simulink model "Laptime_Simulation"  (R2020a)
settings: Solver=VariableStepAuto  StartTime=0.0  StopTime=10.0  RelTol=1e-3
model workspace (MAT data in the model file):
  A = 2
undefined symbols (not defined in the file or in its folder): m_ges
libraries: autolibshared x1
settings Model: Creator=eunde  LastModifiedBy=eunde

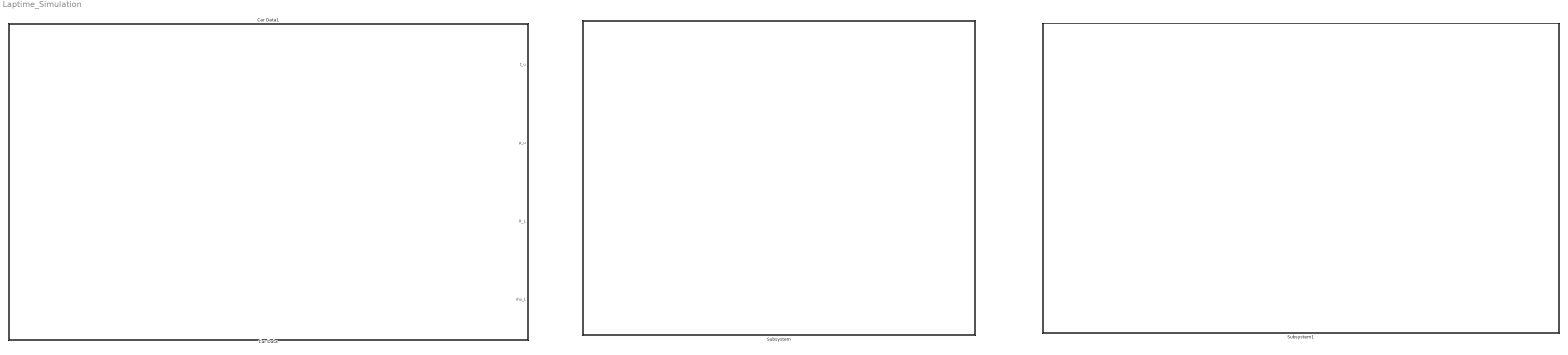
== system Laptime_Simulation ==
  Car Data : Subsystem
  Car Data1 : Subsystem
  Subsystem : Subsystem
  Subsystem1 : Subsystem

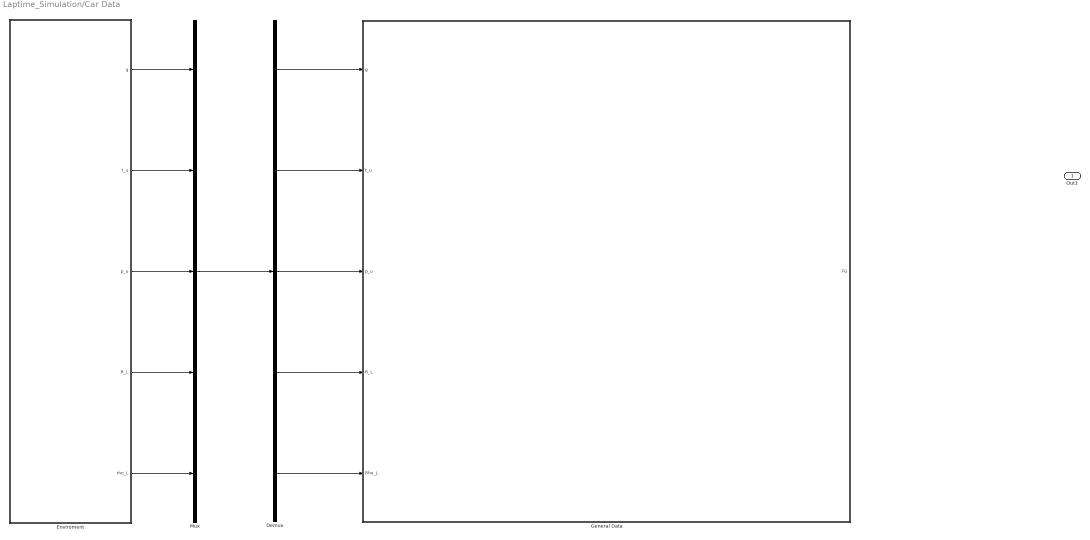
== system Laptime_Simulation/Car Data ==
  Demux : Demux  Outputs=5
  Enviroment : Subsystem
  General Data : Subsystem
  Mux : Mux  Inputs=5
  Out1 : Outport
  wires:
  Enviroment/1(g) -> Mux/1
  Enviroment/2(t_u) -> Mux/2
  Enviroment/3(p_u) -> Mux/3
  Enviroment/4(R_L) -> Mux/4
  Enviroment/5(rho_L) -> Mux/5
  Demux/1 -> General Data/1(g)
  Demux/5 -> General Data/5(Rho_L)
  Mux/1 -> Demux/1
  Demux/2 -> General Data/2(t_u)
  Demux/3 -> General Data/3(p_u)
  Demux/4 -> General Data/4(R_L)

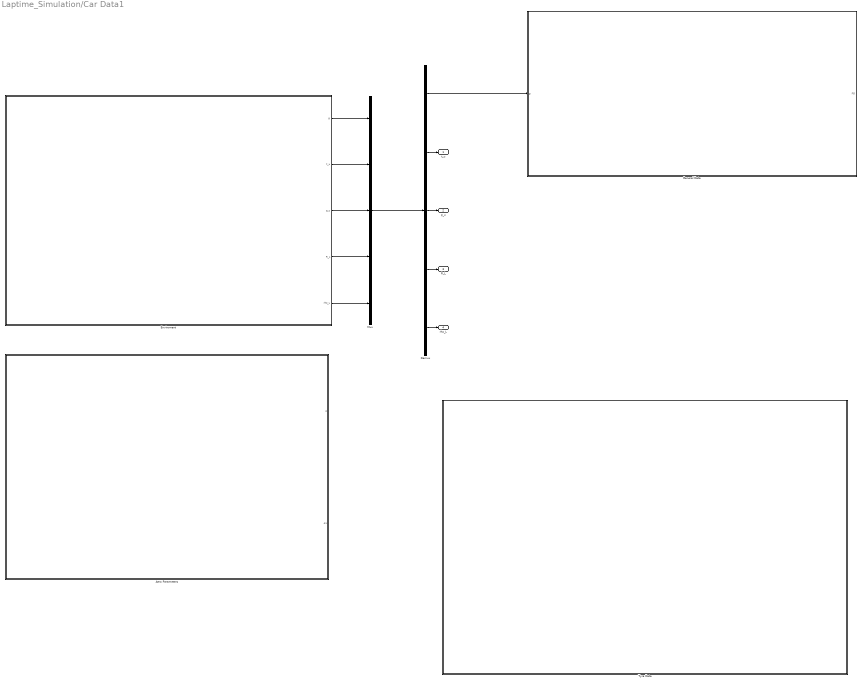
== system Laptime_Simulation/Car Data1 ==
  Aero Parameters : Subsystem
  Demux : Demux  Outputs=5
  Enviroment : Subsystem
  General Data : Subsystem
  Mux : Mux  Inputs=5
  Tyre Data : Subsystem
  t_u : Outport
  p_u : Outport  Port=2
  R_L : Outport  Port=3
  rho_L : Outport  Port=4
  wires:
  Mux/1 -> Demux/1
  Demux/1 -> General Data/1(g)
  Enviroment/5(rho_L) -> Mux/5
  Enviroment/4(R_L) -> Mux/4
  Enviroment/3(p_u) -> Mux/3
  Enviroment/2(t_u) -> Mux/2
  Enviroment/1(g) -> Mux/1
  Demux/2 -> t_u/1
  Demux/3 -> p_u/1
  Demux/4 -> R_L/1
  Demux/5 -> rho_L/1

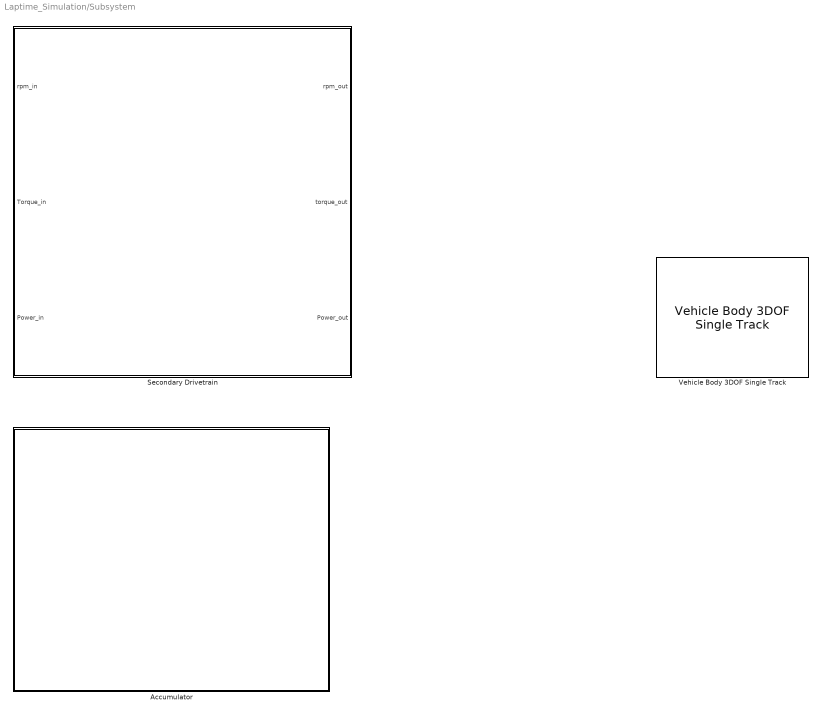
== system Laptime_Simulation/Subsystem ==
  Accumulator : Subsystem
  "Secondary Drivetrain " : Subsystem
  Vehicle Body 3DOF Single Track : autolibshared/Vehicle Body 3DOF Single Track  trackMode=Single (bicycle)  inputMode=External longitudinal velocity  frontSteerMode=on  rearSteerMode=off  windMode=off  muMode=off  extFMode=off  extMMode=off  extXo=off  extpsio=off  extxdoto=off  extro=off  extYo=off  extTamb=off  extydoto=off  aMode=2  NF=2  NR=2  m=m_ges  a=1.4  b=1.6  h=0.35  X_o=0  xdot_o=0  CalphaMode=off  sigmaMode=on  d=0  w=[1.4,1.4]  Cy_f=12e3  Cy_r=11e3  sigma_f=.1  sigma_r=.1  alpha_f_brk=[-.1 .1]  Cy_f_data=[-9e3 9e3]  alpha_r_brk=[-.1 .1]  Cy_r_data=[-9e3 9e3]  Y_o=0  ydot_o=0  Izz=4000  psi_o=0  r_o=0  Af=A  Cd=.3  Cl=.1  Cpm=.1  beta_w=[0:0.01:0.3]  Cs=[0:0.03:0.9]  Cym=[0:0.01:0.3]  Pabs=101325  Tair=273  g=9.81  mu=1  xdot_tol=.01  Fznom=5000  Fxtire_sat=7e4  Fytire_sat=7e4  longOff=0  latOff=0  vertOff=0  wrapAng=off
      settings: SourceProductBaseCode=PW,MT,VE,VP

== system Laptime_Simulation/Subsystem1 ==

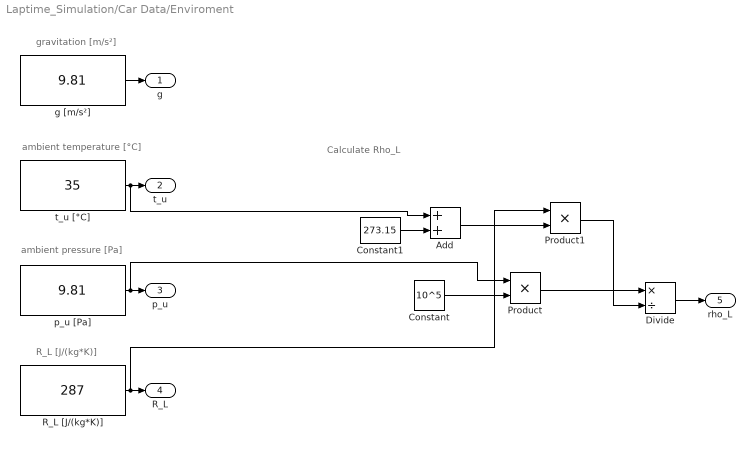
== system Laptime_Simulation/Car Data/Enviroment ==
  note: Calculate Rho_L
  note: gravitation [m/s²]
  note: ambient temperature [°C]
  note: ambient pressure [Pa]
  note: R_L [J/(kg*K)]
  Add : Sum
  Constant : Constant  Value=10^5
  Constant1 : Constant  Value=273.15
  Divide : Product  Inputs=*/
  Product : Product
  Product1 : Product
  R_L [J/(kg*K)] : Constant  Value=287
  g [m/s²] : Constant  Value=9.81
  p_u [Pa] : Constant  Value=9.81
  t_u [°C] : Constant  Value=35
  g : Outport
  t_u : Outport  Port=2
  p_u : Outport  Port=3
  R_L : Outport  Port=4
  rho_L : Outport  Port=5
  wires:
  g [m/s²]/1 -> g/1
  t_u [°C]/1 -> Add/1, t_u/1
  p_u [Pa]/1 -> Product/1, p_u/1
  R_L [J/(kg*K)]/1 -> Product1/1, R_L/1
  Constant/1 -> Product/2
  Product/1 -> Divide/1
  Constant1/1 -> Add/2
  Add/1 -> Product1/2
  Product1/1 -> Divide/2
  Divide/1 -> rho_L/1

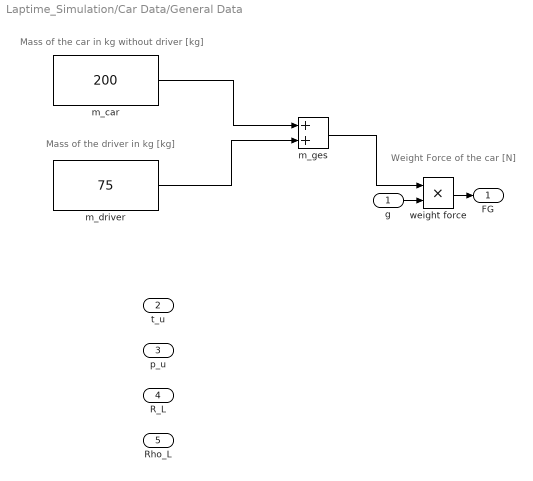
== system Laptime_Simulation/Car Data/General Data ==
  note: Mass of the car in kg without driver [kg]
  note: Mass of the driver in kg [kg]
  note: Weight Force of the car [N]
  g : Inport
  t_u : Inport  Port=2
  p_u : Inport  Port=3
  R_L : Inport  Port=4
  Rho_L : Inport  Port=5
  m_car : Constant  Value=200
  m_driver : Constant  Value=75
  m_ges : Sum
  weight force : Product
  FG : Outport
  wires:
  m_car/1 -> m_ges/1
  m_driver/1 -> m_ges/2
  weight force/1 -> FG/1
  m_ges/1 -> weight force/1
  g/1 -> weight force/2

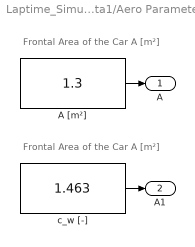
== system Laptime_Simulation/Car Data1/Aero Parameters ==
  note: Frontal Area of the Car A [m²]
  note: Frontal Area of the Car A [m²]
  A [m²] : Constant  Value=1.3
  c_w [-] : Constant  Value=1.463
  A : Outport
  A1 : Outport  Port=2
  wires:
  A [m²]/1 -> A/1
  c_w [-]/1 -> A1/1

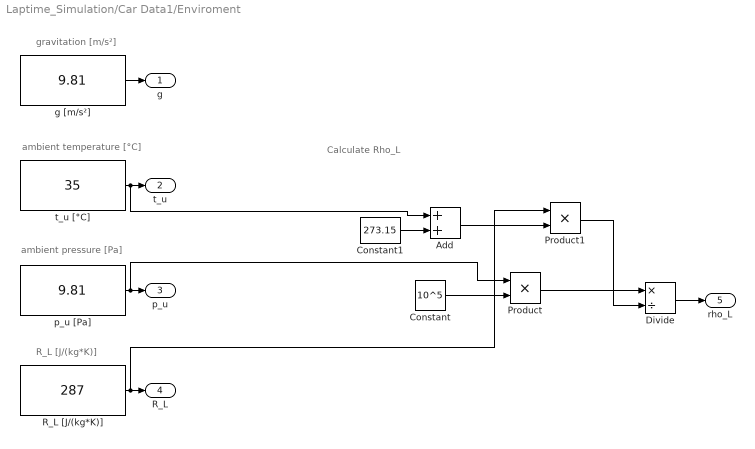
== system Laptime_Simulation/Car Data1/Enviroment ==
  note: R_L [J/(kg*K)]
  note: ambient pressure [Pa]
  note: ambient temperature [°C]
  note: gravitation [m/s²]
  note: Calculate Rho_L
  Add : Sum
  Constant : Constant  Value=10^5
  Constant1 : Constant  Value=273.15
  Divide : Product  Inputs=*/
  Product : Product
  Product1 : Product
  R_L [J/(kg*K)] : Constant  Value=287
  g [m/s²] : Constant  Value=9.81
  p_u [Pa] : Constant  Value=9.81
  t_u [°C] : Constant  Value=35
  g : Outport
  t_u : Outport  Port=2
  p_u : Outport  Port=3
  R_L : Outport  Port=4
  rho_L : Outport  Port=5
  wires:
  Divide/1 -> rho_L/1
  Product1/1 -> Divide/2
  Add/1 -> Product1/2
  Constant1/1 -> Add/2
  Product/1 -> Divide/1
  Constant/1 -> Product/2
  R_L [J/(kg*K)]/1 -> R_L/1, Product1/1
  p_u [Pa]/1 -> p_u/1, Product/1
  t_u [°C]/1 -> t_u/1, Add/1
  g [m/s²]/1 -> g/1

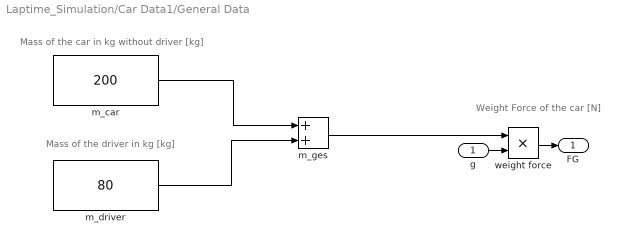
== system Laptime_Simulation/Car Data1/General Data ==
  note: Weight Force of the car [N]
  note: Mass of the driver in kg [kg]
  note: Mass of the car in kg without driver [kg]
  g : Inport
  m_car : Constant  Value=200
  m_driver : Constant  Value=80
  m_ges : Sum
  weight force : Product
  FG : Outport
  wires:
  g/1 -> weight force/2
  m_ges/1 -> weight force/1
  weight force/1 -> FG/1
  m_driver/1 -> m_ges/2
  m_car/1 -> m_ges/1

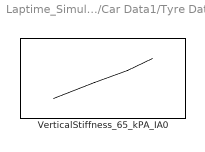
== system Laptime_Simulation/Car Data1/Tyre Data ==
  VerticalStiffness_65_kPA_IA0 : Lookup_n-D  NumberOfTableDimensions=1  BreakpointsForDimension1=[500,600,700,800,900,1000,1100,1200,1300,1400,1500,1600]  Table=[73000,75000,77000,80000,83000,86000,89000,93000,97000,102000,106000,111000]  InternalRulePriority=Speed  RndMeth=Simplest  InputSameDT=on

== system Laptime_Simulation/Subsystem/Accumulator ==
  Accumulator Parameters : Subsystem

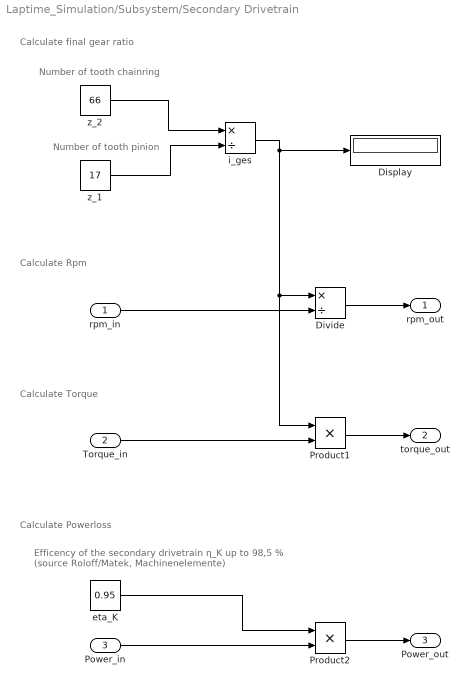
== system Laptime_Simulation/Subsystem/Secondary Drivetrain  ==
  note: Calculate Torque
  note: Calculate Rpm
  note: Calculate final gear ratio
  note: Number of tooth pinion
  note: Number of tooth chainring
  note: Efficency of the secondary drivetrain η_K
      | up to 98,5 % (source Roloff/Matek, Machinenelemente)
  note: Calculate Powerloss
  rpm_in : Inport
  Torque_in : Inport  Port=2
  Power_in : Inport  Port=3
  Display : Display
  Divide : Product  Inputs=*/
  Product1 : Product
  Product2 : Product
  eta_K : Constant  Value=0.95
  i_ges : Product  Inputs=*/
  z_1 : Constant  Value=17
  z_2 : Constant  Value=66
  rpm_out : Outport
  torque_out : Outport  Port=2
  Power_out : Outport  Port=3
  wires:
  z_2/1 -> i_ges/1
  z_1/1 -> i_ges/2
  rpm_in/1 -> Divide/2
  i_ges/1 -> Display/1, Divide/1, Product1/1
  Divide/1 -> rpm_out/1
  Product1/1 -> torque_out/1
  Torque_in/1 -> Product1/2
  eta_K/1 -> Product2/1
  Power_in/1 -> Product2/2
  Product2/1 -> Power_out/1

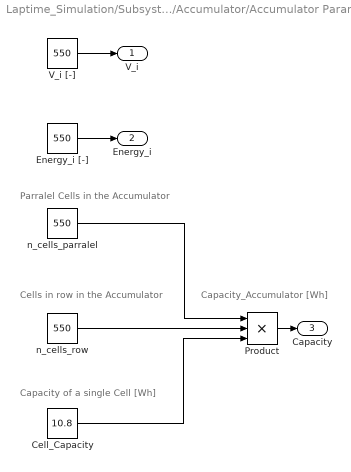
== system Laptime_Simulation/Subsystem/Accumulator/Accumulator Parameters ==
  note: Parralel Cells in the Accumulator
  note: Capacity_Accumulator [Wh]
  note: Cells in row in the Accumulator
  note: Capacity of a single Cell [Wh]
  Cell_Capacity : Constant  Value=10.8
  Energy_i [-] : Constant  Value=550
  Product : Product  Inputs=3
  V_i [-] : Constant  Value=550
  n_cells_parralel : Constant  Value=550
  n_cells_row : Constant  Value=550
  V_i : Outport
  Energy_i : Outport  Port=2
  Capacity : Outport  Port=3
  wires:
  V_i [-]/1 -> V_i/1
  n_cells_row/1 -> Product/2
  Energy_i [-]/1 -> Energy_i/1
  n_cells_parralel/1 -> Product/1
  Product/1 -> Capacity/1
  Cell_Capacity/1 -> Product/3
